simulink library "SDC_coder_lib"  (Simulink 8.6)
settings: Solver=ode45  StartTime=0.0  StopTime=10.0  RelTol=1e-3
undefined symbols (not defined in the file or in its folder): sdc
libraries: dspmtrx3 x8, commsequence2 x6, commcnvcod2 x3, commblkintrlv2 x3, dspbuff3 x3, commdigbbndam3 x2, SDC_coder_lib x1
settings Model: Creator=Kevin  LastModifiedBy=user

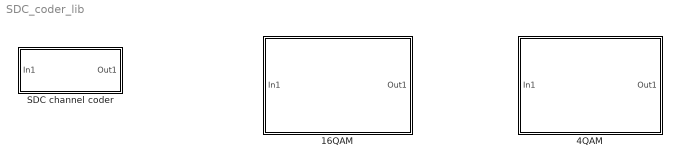
== system SDC_coder_lib ==
  16QAM : Subsystem
  4QAM : Subsystem
  SDC channel coder : Subsystem  BlockChoice=16QAM
      settings: TemplateBlock=self  MemberBlocks=16QAM,4QAM

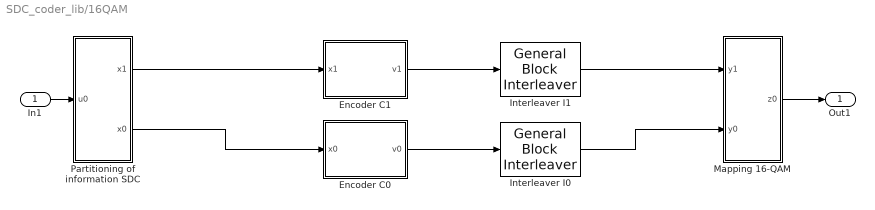
== system SDC_coder_lib/16QAM ==
  In1 : Inport
  Encoder C0 : Subsystem
  Encoder C1 : Subsystem
  Interleaver I0 : commblkintrlv2/General Block Interleaver  permutationVectorSource=Dialog  elements=sdc.interleave_P0
  Interleaver I1 : commblkintrlv2/General Block Interleaver  permutationVectorSource=Dialog  elements=sdc.interleave_P1
  Mapping 16-QAM : Subsystem  AncestorBlock=SDC_coder_lib/16QAM/Mapping 16-QAM
  Partitioning of information SDC : Subsystem
  Out1 : Outport
  wires:
  Partitioning of information SDC/2(x0) -> Encoder C0/1(x0)
  Partitioning of information SDC/1(x1) -> Encoder C1/1(x1)
  Encoder C0/1(v0) -> Interleaver I0/1
  Encoder C1/1(v1) -> Interleaver I1/1
  Interleaver I1/1 -> Mapping 16-QAM/1(y1)
  Interleaver I0/1 -> Mapping 16-QAM/2(y0)
  Mapping 16-QAM/1(z0) -> Out1/1
  In1/1 -> Partitioning of information SDC/1(u0)

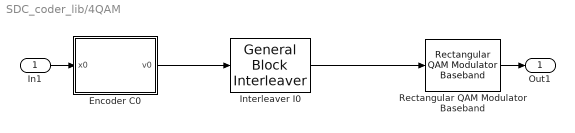
== system SDC_coder_lib/4QAM ==
  In1 : Inport
  Encoder C0 : Subsystem
  Interleaver I0 : commblkintrlv2/General Block Interleaver  elements=sdc.interleave_P0
  Rectangular QAM Modulator Baseband : commdigbbndam3/Rectangular QAM Modulator Baseband  M=SDC_QAM  InType=Bit  Enc=User-defined  Mapping=sdc.qam_map  PowType=Min. distance between symbols  MinDist=sdc.qam_norm  AvgPow=1  PeakPow=1  Ph=0  outDtype=double  outWordLen=16  outUDDataType=sfix(16)  outFracLenMode=Best precision  outFracLen=15
  Out1 : Outport
  wires:
  Interleaver I0/1 -> Rectangular QAM Modulator Baseband/1
  Encoder C0/1(v0) -> Interleaver I0/1
  In1/1 -> Encoder C0/1(x0)
  Rectangular QAM Modulator Baseband/1 -> Out1/1

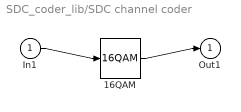
== system SDC_coder_lib/SDC channel coder ==
  In1 : Inport
  16QAM : SDC_coder_lib/16QAM
  Out1 : Outport
  wires:
  In1/1 -> 16QAM/1
  16QAM/1 -> Out1/1

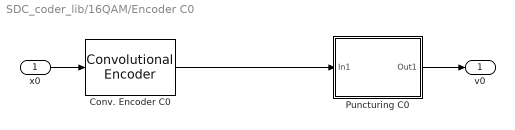
== system SDC_coder_lib/16QAM/Encoder C0 ==
  x0 : Inport
  Conv. Encoder C0 : commcnvcod2/Convolutional Encoder  trellis=conv_poly  opMode=Terminate trellis by appending bits  hasIniStPort=off  hasFinStPort=off  usePuncVector=off  punctureVector=punc_rp35  reset=Unused parameter value
  Puncturing C0 : Subsystem
  v0 : Outport
  wires:
  Puncturing C0/1(Out1) -> v0/1
  x0/1 -> Conv. Encoder C0/1
  Conv. Encoder C0/1 -> Puncturing C0/1(In1)

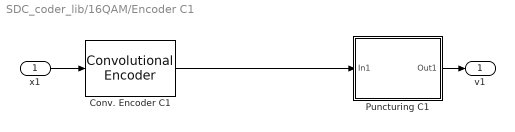
== system SDC_coder_lib/16QAM/Encoder C1 ==
  x1 : Inport
  Conv. Encoder C1 : commcnvcod2/Convolutional Encoder  trellis=conv_poly  opMode=Terminate trellis by appending bits  hasIniStPort=off  hasFinStPort=off  usePuncVector=off  punctureVector=punc_rp35  reset=Unused parameter value
  Puncturing C1 : Subsystem
  v1 : Outport
  wires:
  Puncturing C1/1(Out1) -> v1/1
  x1/1 -> Conv. Encoder C1/1
  Conv. Encoder C1/1 -> Puncturing C1/1(In1)

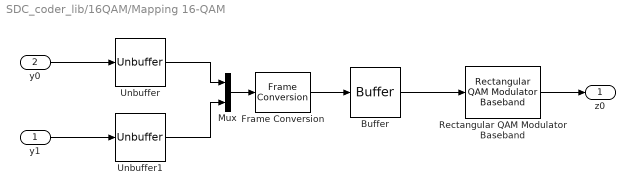
== system SDC_coder_lib/16QAM/Mapping 16-QAM ==
  y1 : Inport
  y0 : Inport  Port=2
  Buffer : dspbuff3/Buffer  N=4*sdc.NmbQAMcells  V=0  ic=0
  Frame Conversion : FrameConversion  InheritSamplingMode=off
  Mux : Mux  Inputs=2
  Rectangular QAM Modulator Baseband : commdigbbndam3/Rectangular QAM Modulator Baseband  M=SDC_QAM  InType=Bit  Enc=User-defined  Mapping=sdc.qam_map  PowType=Min. distance between symbols  MinDist=sdc.qam_norm  AvgPow=1  PeakPow=1  Ph=0  outDtype=double  outWordLen=16  outUDDataType=sfix(16)  outFracLenMode=Best precision  outFracLen=15
  Unbuffer : dspbuff3/Unbuffer  ic=0
  Unbuffer1 : dspbuff3/Unbuffer  ic=0
  z0 : Outport
  wires:
  Rectangular QAM Modulator Baseband/1 -> z0/1
  Mux/1 -> Frame Conversion/1
  Unbuffer1/1 -> Mux/2
  Unbuffer/1 -> Mux/1
  Buffer/1 -> Rectangular QAM Modulator Baseband/1
  Frame Conversion/1 -> Buffer/1
  y0/1 -> Unbuffer/1
  y1/1 -> Unbuffer1/1

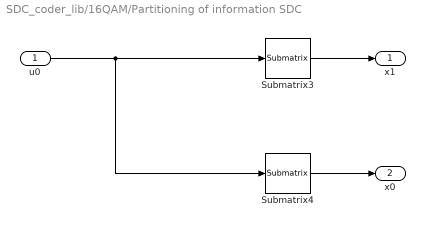
== system SDC_coder_lib/16QAM/Partitioning of information SDC ==
  u0 : Inport
  Submatrix3 : dspmtrx3/Submatrix  RowSpan=Range of rows  RowStartMode=Index  RowStartIndex=sdc.ind_M1  RowEndMode=Last  RowEndIndex=sdc.ind_M1  ColSpan=All columns  ColStartMode=First  ColStartIndex=1  ColEndMode=Last  ColEndIndex=1
  Submatrix4 : dspmtrx3/Submatrix  RowSpan=Range of rows  RowStartMode=First  RowStartIndex=sdc.ind_M0  RowEndMode=Index  RowEndIndex=sdc.ind_M0  ColSpan=All columns  ColStartMode=First  ColStartIndex=1  ColEndMode=Last  ColEndIndex=1
  x1 : Outport
  x0 : Outport  Port=2
  wires:
  Submatrix4/1 -> x0/1
  Submatrix3/1 -> x1/1
  u0/1 -> Submatrix4/1, Submatrix3/1

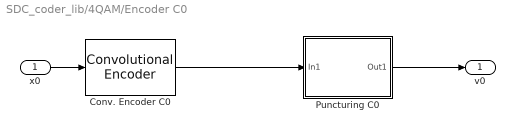
== system SDC_coder_lib/4QAM/Encoder C0 ==
  x0 : Inport
  Conv. Encoder C0 : commcnvcod2/Convolutional Encoder  trellis=conv_poly  opMode=Terminate trellis by appending bits  hasIniStPort=off  hasFinStPort=off  usePuncVector=off  punctureVector=punc_rp35  reset=Unused parameter value
  Puncturing C0 : Subsystem
  v0 : Outport
  wires:
  Puncturing C0/1(Out1) -> v0/1
  x0/1 -> Conv. Encoder C0/1
  Conv. Encoder C0/1 -> Puncturing C0/1(In1)

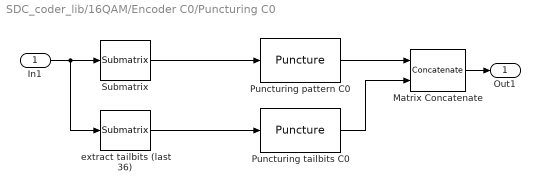
== system SDC_coder_lib/16QAM/Encoder C0/Puncturing C0 ==
  In1 : Inport
  Matrix Concatenate : Concatenate  Mode=Multidimensional array
  Puncturing pattern C0 : commsequence2/Puncture  punctureVector=sdc.punc_pat0
  Puncturing tailbits C0 : commsequence2/Puncture  punctureVector=sdc.punc_tail0
  Submatrix : dspmtrx3/Submatrix  RowSpan=Range of rows  RowStartMode=First  RowStartIndex=1  RowEndMode=Offset from last  RowEndIndex=36  ColSpan=All columns  ColStartMode=First  ColStartIndex=1  ColEndMode=Last  ColEndIndex=1
  extract tailbits (last 36) : dspmtrx3/Submatrix  RowSpan=Range of rows  RowStartMode=Offset from last  RowStartIndex=35  RowEndMode=Last  RowEndIndex=35  ColSpan=All columns  ColStartMode=First  ColStartIndex=1  ColEndMode=Last  ColEndIndex=1
  Out1 : Outport
  wires:
  Matrix Concatenate/1 -> Out1/1
  Puncturing pattern C0/1 -> Matrix Concatenate/1
  Puncturing tailbits C0/1 -> Matrix Concatenate/2
  extract tailbits (last 36)/1 -> Puncturing tailbits C0/1
  Submatrix/1 -> Puncturing pattern C0/1
  In1/1 -> Submatrix/1, extract tailbits (last 36)/1

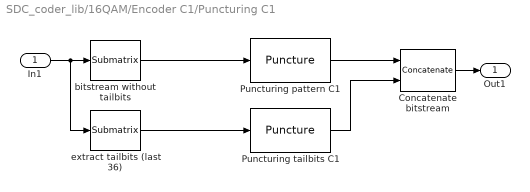
== system SDC_coder_lib/16QAM/Encoder C1/Puncturing C1 ==
  In1 : Inport
  Concatenate bitstream : Concatenate  Mode=Multidimensional array
  Puncturing pattern C1 : commsequence2/Puncture  punctureVector=sdc.punc_pat1
  Puncturing tailbits C1 : commsequence2/Puncture  punctureVector=sdc.punc_tail1
  bitstream without tailbits : dspmtrx3/Submatrix  RowSpan=Range of rows  RowStartMode=First  RowStartIndex=1  RowEndMode=Offset from last  RowEndIndex=36  ColSpan=All columns  ColStartMode=First  ColStartIndex=1  ColEndMode=Last  ColEndIndex=1
  extract tailbits (last 36) : dspmtrx3/Submatrix  RowSpan=Range of rows  RowStartMode=Offset from last  RowStartIndex=35  RowEndMode=Last  RowEndIndex=35  ColSpan=All columns  ColStartMode=First  ColStartIndex=1  ColEndMode=Last  ColEndIndex=1
  Out1 : Outport
  wires:
  Concatenate bitstream/1 -> Out1/1
  In1/1 -> bitstream without tailbits/1, extract tailbits (last 36)/1
  Puncturing pattern C1/1 -> Concatenate bitstream/1
  Puncturing tailbits C1/1 -> Concatenate bitstream/2
  bitstream without tailbits/1 -> Puncturing pattern C1/1
  extract tailbits (last 36)/1 -> Puncturing tailbits C1/1

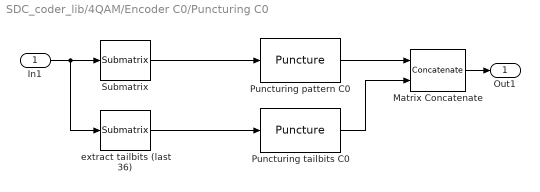
== system SDC_coder_lib/4QAM/Encoder C0/Puncturing C0 ==
  In1 : Inport
  Matrix Concatenate : Concatenate  Mode=Multidimensional array
  Puncturing pattern C0 : commsequence2/Puncture  punctureVector=sdc.punc_pat0
  Puncturing tailbits C0 : commsequence2/Puncture  punctureVector=sdc.punc_tail0
  Submatrix : dspmtrx3/Submatrix  RowSpan=Range of rows  RowStartMode=First  RowStartIndex=1  RowEndMode=Offset from last  RowEndIndex=36  ColSpan=All columns  ColStartMode=First  ColStartIndex=1  ColEndMode=Last  ColEndIndex=1
  extract tailbits (last 36) : dspmtrx3/Submatrix  RowSpan=Range of rows  RowStartMode=Offset from last  RowStartIndex=35  RowEndMode=Last  RowEndIndex=35  ColSpan=All columns  ColStartMode=First  ColStartIndex=1  ColEndMode=Last  ColEndIndex=1
  Out1 : Outport
  wires:
  Matrix Concatenate/1 -> Out1/1
  Puncturing pattern C0/1 -> Matrix Concatenate/1
  Puncturing tailbits C0/1 -> Matrix Concatenate/2
  extract tailbits (last 36)/1 -> Puncturing tailbits C0/1
  Submatrix/1 -> Puncturing pattern C0/1
  In1/1 -> Submatrix/1, extract tailbits (last 36)/1
